simulink model "lab_4"  (R2017b)
settings: Solver=VariableStepAuto  StartTime=0.0  StopTime=10  RelTol=1e-3
settings Model: Creator=kamzab95  LastModifiedBy=kamzab95

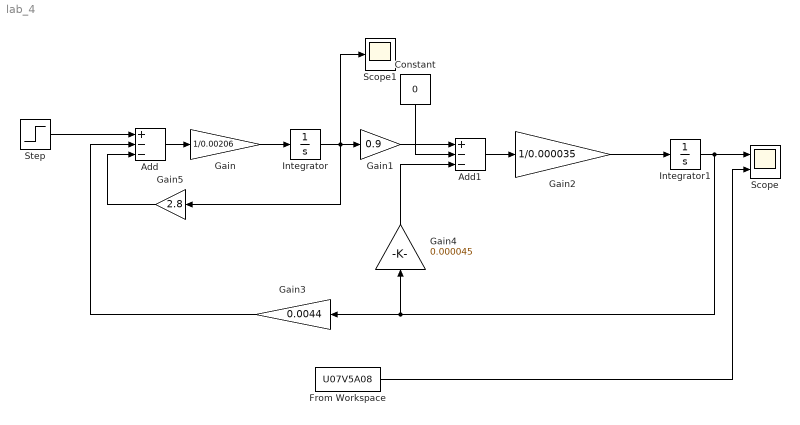
== system lab_4 ==
  Add : Sum  Inputs=+--
  Add1 : Sum  Inputs=+--
  Constant : Constant  Value=0
  From Workspace : FromWorkspace  VariableName=U07V5A08  SampleTime=0
  Gain : Gain  Gain=1/0.00206
  Gain1 : Gain  Gain=0.9
  Gain2 : Gain  Gain=1/0.000035
  Gain3 : Gain  Gain=0.0044
  Gain4 : Gain  Gain=0.000045
  Gain5 : Gain  Gain=2.8
  Integrator : Integrator
  Integrator1 : Integrator
  Scope : Scope  NumInputPorts=2
  Scope1 : Scope
  Step : Step  Time=1.6  After=7.5  SampleTime=0
  wires:
  Step/1 -> Add/1
  Add/1 -> Gain/1
  Gain/1 -> Integrator/1
  Integrator/1 -> Scope1/1, Gain5/1, Gain1/1
  Gain1/1 -> Add1/1
  Add1/1 -> Gain2/1
  Gain2/1 -> Integrator1/1
  Integrator1/1 -> Scope/1, Gain3/1, Gain4/1
  Gain3/1 -> Add/2
  Constant/1 -> Add1/2
  From Workspace/1 -> Scope/2
  Gain5/1 -> Add/3
  Gain4/1 -> Add1/3
